simulink model "piezo_constraint"  (R2021a)
settings: Solver=ode1  StartTime=0.0  StopTime=inf  FixedStep=0.001  RelTol=1e-3
PostLoadFcn:
  | , if any(exist('dsrtsu_mdlpostloadfcn', 'file') ~= 0), dsrtsu_mdlpostloadfcn('Execute', bdroot); end,
InitFcn:
  | , if any(exist('rtifpga_mdlclblib', 'file') ~= 0), rtifpga_mdlclblib('Init', bdroot); end,
libraries: simulink x3, rti1202lib_adc_class1 x2, rti1202lib_dac_class1 x1
Description:
  | Standard RTI1202 template.
  | Supported MATLAB version:  R2021a.
settings Model: Tag=RTI1202  DSRTSU_INTERNAL_RTI_VER=610  DSRTSU_INTERNAL_RTI_TYPE=rti1202  RTICANMMDATA=struct('GeneralSetupData',struct('modelroot','C:\Users\VM-User\Desktop\MigrationScripts','generalsettings',struct('filesettings',struct('destfolder',struct('Name','RTICANMM_FILES','Check',1),'buildfolder',struct('Name','.','Check',1),'AbsDestfolder',struct('Name','C:\Users\VM-User\Desktop\MigrationScripts\RTICANMM_FILES'),'AbsBuildfolder',struct('Name','C:\Users\VM-User\Desktop\MigrationScripts'))),'options',struct('addpaths',1,'rmpaths',1,'addtrcexclusion',true,'cannavigator',struct('checkmonitoring',0),'show_usrtrc',0,'use_usrtrc',0),'advanced',struct('options',ones(1,100)),'MPSetup',{{}},'RTI',struct('Type','RTI1202','Ver','7.17','Date','02-Nov-2021'),'modelname','','block','untitled'))  DSRTSU_INTERNAL_RTIFPGA=200  DSRTSU_INTERNAL_RTISTBM_VER=22.2  PacingRate=0.010000  Creator=217_03  LastModifiedBy=217_03
settings SolverCC: AlgebraicLoopSolver=TrustRegion
settings DataIOCC: ReturnWorkspaceOutputs=off
settings OptimizationCC: BlockReduction=off  ConditionallyExecuteInputs=off  OptimizeBlockIOStorage=off  BufferReuse=off  GlobalBufferReuse=off  ExpressionFolding=off  LocalBlockOutputs=off  OptimizeDataStoreBuffers=off  BusAssignmentInplaceUpdate=off
settings DebuggingCC: PregeneratedLibrarySubsystemCodeDiagnostic=none  SFMachineParentedDataDiag=warning  ArithmeticOperatorsInVariantConditions=warning
settings HardwareCC: ProdBitPerPointer=32  ProdBitPerSizeT=32  ProdBitPerPtrDiffT=32  ProdLargestAtomicInteger=Integer  ProdEndianess=BigEndian  ProdWordSize=32  ProdLongLongMode=on  ProdHWDeviceType=Custom Processor->Custom  TargetIntDivRoundTo=Zero  TargetEndianess=BigEndian  TargetHWDeviceType=Custom Processor->Custom
settings ModelReferenceCC: EnableParallelModelReferenceBuilds=on  ParallelModelReferenceMATLABWorkerInit=Load Top Model
settings SFSimCC: SimUseLocalCustomCode=off  MATLABDynamicMemAlloc=off  CustomCodeUndefinedFunction=UseInterfaceOnly
settings RTWCC: Description=dSPACE DS1202 Hardware Platform  SystemTargetFile=rti1202.tlc  MakeCommand=make_rti  TemplateMakefile=rti1202.tmf  RTWUseLocalCustomCode=off
settings CodeAppCC: StateflowObjectComments=on
settings STFCustomTargetCC: ParMdlRefBuildCompliant=on  GRTInterface=off  UseToolchainInfoCompliant=off  SystemTargetFile=rti1202.tlc
settings GRTTargetCC: TargetLangStandard=C89/C90 (ANSI)  CompOptLevelCompliant=off  ConcurrentExecutionCompliant=off  CombineOutputUpdateFcns=off  MatFileLogging=off  CPPClassGenCompliant=off  UseToolchainInfoCompliant=off
settings ConfigComp: CovMetricSettings=dswe

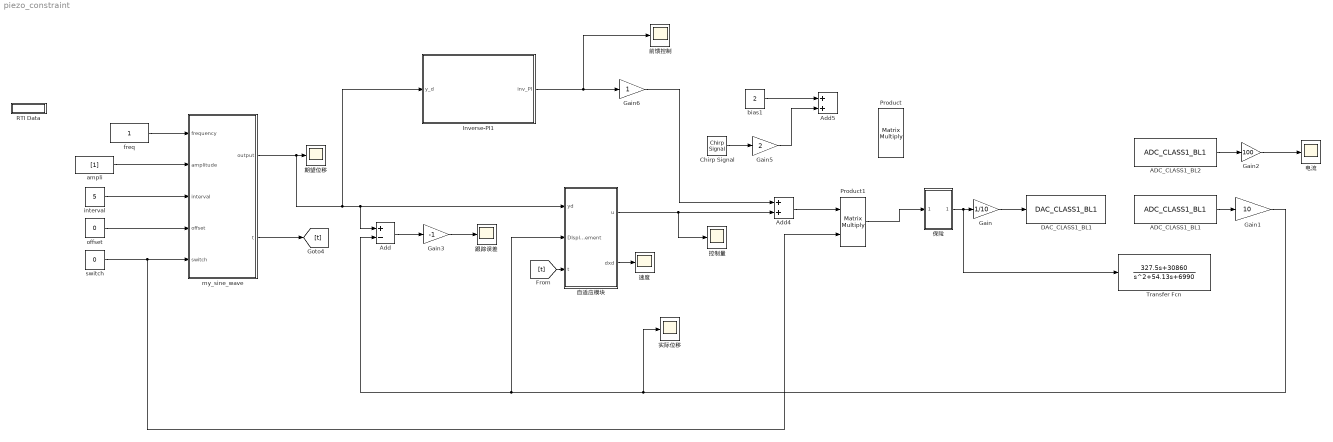
== system piezo_constraint ==
  ADC_CLASS1_BL1 : rti1202lib_adc_class1/ADC_CLASS1_BL1  DSProperties=struct('RTI',struct('Version',uint32(1),'BlockType',struct('isSLSource',uint8(1),'isSLSink',uint8(1),'isHWSource',uint8(0),'isHWSink',uint8(1),'isSetup',uint8(0),'isInline',uint8(1),'isNonInline',uint8(0),'isInterrupt',uint8(0),'isChannelwise',uint8(1)),'IOBoardType',{{'DS120X','STD','ADCC1'}},'UnitType','ADC','Identifier','ADC','DialogType','ML','BlockSet','NONE','SlaveProcessor','NONE'))  RTIBlockInterface=struct('InputPortsActive',0,'InputPortsWidth',int32(1),'InputPortsDataType',{{'SS_BOOLEAN'}},'InputPortsName',{{'Continue'}},'OutputPortsActive',[1 0],'OutputPortsWidth',int32([1 1]),'OutputPortsDataType',{{'SS_DOUBLE','SS_INT16'}},'OutputPortsName',{{'ADC','Status'}},'DialogFcn','rti120xstdadcc1adcgui','SampleTime',{{-1}},'InitLevel',3,'IconTransparency','on','BlockDisplay',{{['ADC CL1\nChannel: 10'],'center'}},'BlockName',struct('Token',{{'ADC_CLASS1_BL1'}}))  RTIBlockParameters=struct('ReadMode',{{1,'OFF',[1 2]}},'ChannelNo',{{10,'OFF',[]}},'ConversionMode',{{1,'OFF',[1 2]}},'TriggerSource',{{1,'OFF',[1 2]}},'TriggerLineIn',{{1,'OFF',[1 16]}},'SampleMode',{{1,'OFF',[1 2]}},'BurstTriggerSource',{{1,'OFF',[1 2]}},'BurstTriggerLine',{{1,'OFF',[1 16]}},'ConvTriggerSource',{{3,'OFF',[1 3]}},'ConvTriggerLine',{{1,'OFF',[1 16]}},'ConvPeriod',{{'100e-6','OFF',[1e-6 1.34]}},'ConvPeriodCheck',{{0,'OFF',[]}},'BurstSize',{{'10','OFF',[]}},'BurstSizeCheck',{{0,'OFF',[]}},'DataSetOffset',{{'0','OFF',[]}},'DataSetOffsetCheck',{{0,'OFF',[]}},'DataSetLength',{{'1','OFF',[]}},'DataSetLengthCheck',{{0,'OFF',[]}},'EnableTriggerEvent',{{0,'OFF',[0 1]}},'TriggerMode',{{2,'OFF',[1 3]}},'TriggerLineOut',{{1,'OFF',[1 16]}},'ADCSWStartEnable',{{0,'OFF',[0 1]}},'SampleTime',{{'-1','OFF',[-1 inf]}},'SampleTimeCheck',{{1,'OFF',[]}},'StatusPortEnable',{{0,'OFF',[0 1]}},'TLCFileName',{{'rti120xadc_c1_adc','OFF',[]}})  RTISFcnParameters=struct('ReadMode','int16','ChannelNo','int16','ConversionMode','int16','TriggerSource','int16','TriggerLineIn','int16','SampleMode','int16','BurstTriggerSource','int16','BurstTriggerLine','int16','ConvTriggerSource','int16','ConvTriggerLine','int16','ConvPeriod','double','BurstSize','int16','DataSetOffset','int16','DataSetLength','int16','EnableTriggerEvent','int16','TriggerMode','int16','TriggerLineOut','int16','ADCSWStartEnable','int16','SampleTime','double','StatusPortEnable','int16','TLCFileName','char')  RTIBlockParaDefault=struct('ReadMode',1,'ChannelNo',1,'ConversionMode',1,'TriggerSource',1,'TriggerLineIn',1,'SampleMode',1,'BurstTriggerSource',1,'BurstTriggerLine',1,'ConvTriggerSource',3,'ConvTriggerLine',1,'ConvPeriod',0.0001,'ConvPeriodCheck',0,'BurstSize',10,'BurstSizeCheck',0,'DataSetOffset',0,'DataSetOffsetCheck',0,'DataSetLength',1,'DataSetLengthCheck',0,'EnableTriggerEvent',0,'TriggerMode',2,'TriggerLineOut',1,'ADCSWStartEnable',0,'SampleTime',-1,'SampleTimeCheck',1,'StatusPortEnable',0,'TLCFileName','rti120xadc_c1_adc')
  ADC_CLASS1_BL2 : rti1202lib_adc_class1/ADC_CLASS1_BL1  DSProperties=struct('RTI',struct('Version',uint32(1),'BlockType',struct('isSLSource',uint8(1),'isSLSink',uint8(1),'isHWSource',uint8(0),'isHWSink',uint8(1),'isSetup',uint8(0),'isInline',uint8(1),'isNonInline',uint8(0),'isInterrupt',uint8(0),'isChannelwise',uint8(1)),'IOBoardType',{{'DS120X','STD','ADCC1'}},'UnitType','ADC','Identifier','ADC','DialogType','ML','BlockSet','NONE','SlaveProcessor','NONE'))  RTIBlockInterface=struct('InputPortsActive',0,'InputPortsWidth',int32(1),'InputPortsDataType',{{'SS_BOOLEAN'}},'InputPortsName',{{'Continue'}},'OutputPortsActive',[1 0],'OutputPortsWidth',int32([1 1]),'OutputPortsDataType',{{'SS_DOUBLE','SS_INT16'}},'OutputPortsName',{{'ADC','Status'}},'DialogFcn','rti120xstdadcc1adcgui','SampleTime',{{-1}},'InitLevel',3,'IconTransparency','on','BlockDisplay',{{['ADC CL1\nChannel: 13'],'center'}},'BlockName',struct('Token',{{'ADC_CLASS1_BL1'}}))  RTIBlockParameters=struct('ReadMode',{{1,'OFF',[1 2]}},'ChannelNo',{{13,'OFF',[]}},'ConversionMode',{{1,'OFF',[1 2]}},'TriggerSource',{{1,'OFF',[1 2]}},'TriggerLineIn',{{1,'OFF',[1 16]}},'SampleMode',{{1,'OFF',[1 2]}},'BurstTriggerSource',{{1,'OFF',[1 2]}},'BurstTriggerLine',{{1,'OFF',[1 16]}},'ConvTriggerSource',{{3,'OFF',[1 3]}},'ConvTriggerLine',{{1,'OFF',[1 16]}},'ConvPeriod',{{'100e-6','OFF',[1e-6 1.34]}},'ConvPeriodCheck',{{0,'OFF',[]}},'BurstSize',{{'10','OFF',[]}},'BurstSizeCheck',{{0,'OFF',[]}},'DataSetOffset',{{'0','OFF',[]}},'DataSetOffsetCheck',{{0,'OFF',[]}},'DataSetLength',{{'1','OFF',[]}},'DataSetLengthCheck',{{0,'OFF',[]}},'EnableTriggerEvent',{{0,'OFF',[0 1]}},'TriggerMode',{{2,'OFF',[1 3]}},'TriggerLineOut',{{1,'OFF',[1 16]}},'ADCSWStartEnable',{{0,'OFF',[0 1]}},'SampleTime',{{'-1','OFF',[-1 inf]}},'SampleTimeCheck',{{1,'OFF',[]}},'StatusPortEnable',{{0,'OFF',[0 1]}},'TLCFileName',{{'rti120xadc_c1_adc','OFF',[]}})  RTISFcnParameters=struct('ReadMode','int16','ChannelNo','int16','ConversionMode','int16','TriggerSource','int16','TriggerLineIn','int16','SampleMode','int16','BurstTriggerSource','int16','BurstTriggerLine','int16','ConvTriggerSource','int16','ConvTriggerLine','int16','ConvPeriod','double','BurstSize','int16','DataSetOffset','int16','DataSetLength','int16','EnableTriggerEvent','int16','TriggerMode','int16','TriggerLineOut','int16','ADCSWStartEnable','int16','SampleTime','double','StatusPortEnable','int16','TLCFileName','char')  RTIBlockParaDefault=struct('ReadMode',1,'ChannelNo',1,'ConversionMode',1,'TriggerSource',1,'TriggerLineIn',1,'SampleMode',1,'BurstTriggerSource',1,'BurstTriggerLine',1,'ConvTriggerSource',3,'ConvTriggerLine',1,'ConvPeriod',0.0001,'ConvPeriodCheck',0,'BurstSize',10,'BurstSizeCheck',0,'DataSetOffset',0,'DataSetOffsetCheck',0,'DataSetLength',1,'DataSetLengthCheck',0,'EnableTriggerEvent',0,'TriggerMode',2,'TriggerLineOut',1,'ADCSWStartEnable',0,'SampleTime',-1,'SampleTimeCheck',1,'StatusPortEnable',0,'TLCFileName','rti120xadc_c1_adc')
  Add : Sum  Inputs=+-
  Add4 : Sum
  Add5 : Sum
  Chirp Signal : simulink/Sources/Chirp Signal  f1=1  T=20  f2=50
  DAC_CLASS1_BL1 : rti1202lib_dac_class1/DAC_CLASS1_BL1  DSProperties=struct('RTI',struct('Version',uint32(2),'BlockType',struct('isSLSource',uint8(0),'isSLSink',uint8(1),'isHWSource',uint8(0),'isHWSink',uint8(1),'isSetup',uint8(0),'isInline',uint8(1),'isNonInline',uint8(0),'isInterrupt',uint8(0),'isChannelwise',uint8(1)),'IOBoardType',{{'DS120X','STD','DACC1'}},'UnitType','DAC','Identifier','DAC','DialogType','ML','BlockSet','NONE','SlaveProcessor','NONE'))  RTIBlockInterface=struct('InputPortsActive',1,'InputPortsWidth',int32(1),'InputPortsDataType',{{'SS_DOUBLE'}},'InputPortsName',{{['DAC 5']}},'DialogFcn','rti120xstddacc1dacgui','InitLevel',3,'IconTransparency','on','BlockDisplay',{{['DAC CL1\nChannel: 5'],'center'}},'BlockName',struct('Token',{{'DAC_CLASS1_BL1'}}))  RTIBlockParameters=struct('ChannelNo',{{5,'OFF',[]}},'ChannelNumOf',{{1,'OFF',[]}},'InitialValue1',{{'0','OFF',[-10 10]}},'InitialValue2',{{'0','OFF',[-10 10]}},'InitialValue3',{{'0','OFF',[-10 10]}},'InitialValue4',{{'0','OFF',[-10 10]}},'InitialValue5',{{'0','OFF',[-10 10]}},'InitialValue6',{{'0','OFF',[-10 10]}},'InitialValue7',{{'0','OFF',[-10 10]}},'InitialValue8',{{'0','OFF',[-10 10]}},'InitialValue9',{{'0','OFF',[-10 10]}},'InitialValue10',{{'0','OFF',[-10 10]}},'InitialValue11',{{'0','OFF',[-10 10]}},'InitialValue12',{{'0','OFF',[-10 10]}},'InitialValue13',{{'0','OFF',[-10 10]}},'InitialValue14',{{'0','OFF',[-10 10]}},'InitialValue15',{{'0','OFF',[-10 10]}},'InitialValue16',{{'0','OFF',[-10 10]}},'OutputMode',{{ones(1,16),'OFF',[1 2]}},'TermValue1',{{'0','OFF',[-10 10]}},'TermValue2',{{'0','OFF',[-10 10]}},'TermValue3',{{'0','OFF',[-10 10]}},'TermValue4',{{'0','OFF',[-10 10]}},'TermValue5',{{'0','OFF',[-10 10]}},'TermValue6',{{'0','OFF',[-10 10]}},'TermValue7',{{'0','OFF',[-10 10]}},'TermValue8',{{'0','OFF',[-10 10]}},'TermValue9',{{'0','OFF',[-10 10]}},'TermValue10',{{'0','OFF',[-10 10]}},'TermValue11',{{'0','OFF',[-10 10]}},'TermValue12',{{'0','OFF',[-10 10]}},'TermValue13',{{'0','OFF',[-10 10]}},'TermValue14',{{'0','OFF',[-10 10]}},'TermValue15',{{'0','OFF',[-10 10]}},'TermValue16',{{'0','OFF',[-10 10]}},'EnableTermMode',{{0,'OFF',[0 1]}},'TLCFileName',{{'rti120xdac_c1_dac','OFF',[]}},'InitialValueBuildCheck1',{{0,'OFF',[]}},'InitialValueBuildCheck2',{{0,'OFF',[]}},'InitialValueBuildCheck3',{{0,'OFF',[]}},'InitialValueBuildCheck4',{{0,'OFF',[]}},'InitialValueBuildCheck5',{{1,'OFF',[]}},'InitialValueBuildCheck6',{{0,'OFF',[]}},'InitialValueBuildCheck7',{{0,'OFF',[]}},'InitialValueBuildCheck8',{{0,'OFF',[]}},'InitialValueBuildCheck9',{{0,'OFF',[]}},'InitialValueBuildCheck10',{{0,'OFF',[]}},'InitialValueBuildCheck11',{{0,'OFF',[]}},'InitialValueBuildCheck12',{{0,'OFF',[]}},'InitialValueBuildCheck13',{{0,'OFF',[]}},'InitialValueBuildCheck14',{{0,'OFF',[]}},'InitialValueBuildCheck15',{{0,'OFF',[]}},'InitialValueBuildCheck16',{{0,'OFF',[]}},'TermValueBuildCheck1',{{0,'OFF',[]}},'TermValueBuildCheck2',{{0,'OFF',[]}},'TermValueBuildCheck3',{{0,'OFF',[]}},'TermValueBuildCheck4',{{0,'OFF',[]}},'TermValueBuildCheck5',{{0,'OFF',[]}},'TermValueBuildCheck6',{{0,'OFF',[]}},'TermValueBuildCheck7',{{0,'OFF',[]}},'TermValueBuildCheck8',{{0,'OFF',[]}},'TermValueBuildCheck9',{{0,'OFF',[]}},'TermValueBuildCheck10',{{0,'OFF',[]}},'TermValueBuildCheck11',{{0,'OFF',[]}},'TermValueBuildCheck12',{{0,'OFF',[]}},'TermValueBuildCheck13',{{0,'OFF',[]}},'TermValueBuildCheck14',{{0,'OFF',[]}},'TermValueBuildCheck15',{{0,'OFF',[]}},'TermValueBuildCheck16',{{0,'OFF',[]}})  RTISFcnParameters=struct('ChannelNo','int16','ChannelNumOf','int16','InitialValue1','double','InitialValue2','double','InitialValue3','double','InitialValue4','double','InitialValue5','double','InitialValue6','double','InitialValue7','double','InitialValue8','double','InitialValue9','double','InitialValue10','double','InitialValue11','double','InitialValue12','double','InitialValue13','double','InitialValue14','double','InitialValue15','double','InitialValue16','double','OutputMode','int16','TermValue1','double','TermValue2','double','TermValue3','double','TermValue4','double','TermValue5','double','TermValue6','double','TermValue7','double','TermValue8','double','TermValue9','double','TermValue10','double','TermValue11','double','TermValue12','double','TermValue13','double','TermValue14','double','TermValue15','double','TermValue16','double','EnableTermMode','int16','TLCFileName','char')  RTIBlockParaDefault=struct('ChannelNo',1,'ChannelNumOf',1,'InitialValue1',0,'InitialValue2',0,'InitialValue3',0,'InitialValue4',0,'InitialValue5',0,'InitialValue6',0,'InitialValue7',0,'InitialValue8',0,'InitialValue9',0,'InitialValue10',0,'InitialValue11',0,'InitialValue12',0,'InitialValue13',0,'InitialValue14',0,'InitialValue15',0,'InitialValue16',0,'OutputMode',ones(1,16),'TermValue1',0,'TermValue2',0,'TermValue3',0,'TermValue4',0,'TermValue5',0,'TermValue6',0,'TermValue7',0,'TermValue8',0,'TermValue9',0,'TermValue10',0,'TermValue11',0,'TermValue12',0,'TermValue13',0,'TermValue14',0,'TermValue15',0,'TermValue16',0,'EnableTermMode',0,'TLCFileName','rti120xdac_c1_dac','InitialValueBuildCheck1',0,'InitialValueBuildCheck2',0,'InitialValueBuildCheck3',0,'InitialValueBuildCheck4',0,'InitialValueBuildCheck5',0,'InitialValueBuildCheck6',0,'InitialValueBuildCheck7',0,'InitialValueBuildCheck8',0,'InitialValueBuildCheck9',0,'InitialValueBuildCheck10',0,'InitialValueBuildCheck11',0,'InitialValueBuildCheck12',0,'InitialValueBuildCheck13',0,'InitialValueBuildCheck14',0,'InitialValueBuildCheck15',0,'InitialValueBuildCheck16',0,'TermValueBuildCheck1',0,'TermValueBuildCheck2',0,'TermValueBuildCheck3',0,'TermValueBuildCheck4',0,'TermValueBuildCheck5',0,'TermValueBuildCheck6',0,'TermValueBuildCheck7',0,'TermValueBuildCheck8',0,'TermValueBuildCheck9',0,'TermValueBuildCheck10',0,'TermValueBuildCheck11',0,'TermValueBuildCheck12',0,'TermValueBuildCheck13',0,'TermValueBuildCheck14',0,'TermValueBuildCheck15',0,'TermValueBuildCheck16',0)
  Gain : Gain  Gain=1/10
  Gain1 : Gain  Gain=10
  Gain2 : Gain  Gain=100
  Gain3 : Gain  Gain=-1
  Gain5 : Gain  Gain=2
  Gain6 : Gain
  Inverse-PI1 : Subsystem
  Product : Product  Multiplication=Matrix(*)  OutDataTypeStr=double
  Product1 : Product  Multiplication=Matrix(*)  OutDataTypeStr=double
  RTI Data : Subsystem  Tag=struct('RTIDataServer',struct('RTIDataServerVs','2','RTIModelDescription','struct(''main'',''piezo_constraint_huheyu'',''sub'','''',''isMp'',0)'))  LoadFcn="if exist('rtidc'), try,  rtidc('DataHostBlockClbLoad', gcbh); catch, disp(['Warning: ''LoadFcn'' for RTI Data block failed: ' lasterr]); end, end,"  mask(RTI_DATA_HOST){}
      mask help:
      | RTI Data Block.
      | This block is used by RTI to store internal model-dependent data.
      | Please keep this block on the root level of the model. Deleting this block will result in data loss.
      |
      | NEVER DELETE OR COPY THIS BLOCK!
      settings: CopyFcn="if exist('rtidc'), try,  rtidc('DataHostBlockClbCopy', gcbh); catch, disp(['Warning: ''CopyFcn'' for RTI Data block failed: ' lasterr]); end, end,"  DeleteFcn="if exist('rtidc'), try,  rtidc('DataHostBlockClbDelete', gcbh); catch, disp(['Warning: ''DeleteFcn'' for RTI Data block failed: ' lasterr]); end, end,"  ModelCloseFcn="if exist('rtidc'), try,  rtidc('DataHostBlockClbModelClose', gcbh); catch, disp(['Warning: ''ModelCloseFcn'' for RTI Data block failed: ' lasterr]); end, end,"  PreSaveFcn="if exist('rtidc'), try,  rtidc('DataHostBlockClbPreSave', gcbh); catch, disp(['Warning: ''PreSaveFcn'' for RTI Data block failed: ' lasterr]); end, end,"  PostSaveFcn="if exist('rtidc'), try,  rtidc('DataHostBlockClbPostSave', gcbh); catch, disp(['Warning: ''PostSaveFcn'' for RTI Data block failed: ' lasterr]); end, end,"  NameChangeFcn="if exist('rtidc'), try,  rtidc('DataHostBlockClbNameChange', gcbh); catch, disp(['Warning: ''NameChangeFcn'' for RTI Data block failed: ' lasterr]); end, end,"
      mask Help:
      | RTI Data Block.
      | This block is used by RTI to store internal model-dependent data.
      | Please keep this block on the root level of the model. Deleting this block will result in data loss.
      | 
      | NEVER DELETE OR COPY THIS BLOCK!
      mask Display:
      | text(0.5, 0.5, 'RTI Data', 'HorizontalAlignment', 'center');
      | plot([1 0]);
  Transfer Fcn : TransferFcn  Numerator=[327.5 30860]  Denominator=[1 54.13 6990]
  ampli : Constant  Value=[1]
  bias1 : Constant  Value=2
  freq : Constant
  interval : Constant  Value=5
  my_sine_wave : Subsystem
  offset : Constant  Value=0
  switch : Constant  Value=0  OutMin=[0]  OutMax=[1]  OutDataTypeStr=int8
  保险 : Subsystem
  前馈控制 : Scope
  实际位移 : Scope
  控制量 : Scope
  期望位移 : Scope
  电流 : Scope
  自适应模块 : Subsystem
  跟踪误差 : Scope
  速度 : Scope
  wires:
  ampli/1 -> my_sine_wave/2(amplitude)
  interval/1 -> my_sine_wave/3(interval)
  ADC_CLASS1_BL1/1 -> Gain1/1
  Gain/1 -> DAC_CLASS1_BL1/1
  保险/1(Out2) -> Transfer Fcn/1, Gain/1
  my_sine_wave/1(output) -> Inverse-PI1/1(y_d), 自适应模块/1(yd), Add/1, 期望位移/1
  ADC_CLASS1_BL2/1 -> Gain2/1
  Gain2/1 -> 电流/1
  Inverse-PI1/1(inv_PI) -> 前馈控制/1, Gain6/1
  Chirp Signal/1 -> Gain5/1
  bias1/1 -> Add5/1
  Gain5/1 -> Add5/2
  Gain6/1 -> Add4/1
  my_sine_wave/2(t) -> [t]
  switch/1 -> Product1/2, my_sine_wave/5(switch)
  offset/1 -> my_sine_wave/4(offset)
  freq/1 -> my_sine_wave/1(frequency)
  Product1/1 -> 保险/1(In1)
  自适应模块/1(u) -> 控制量/1, Add4/2
  Add4/1 -> Product1/1
  [t] -> 自适应模块/3(t)
  Gain1/1 -> 实际位移/1, 自适应模块/2(DIsplacement), Add/2
  Gain3/1 -> 跟踪误差/1
  Add/1 -> Gain3/1
  自适应模块/2(dxd) -> 速度/1

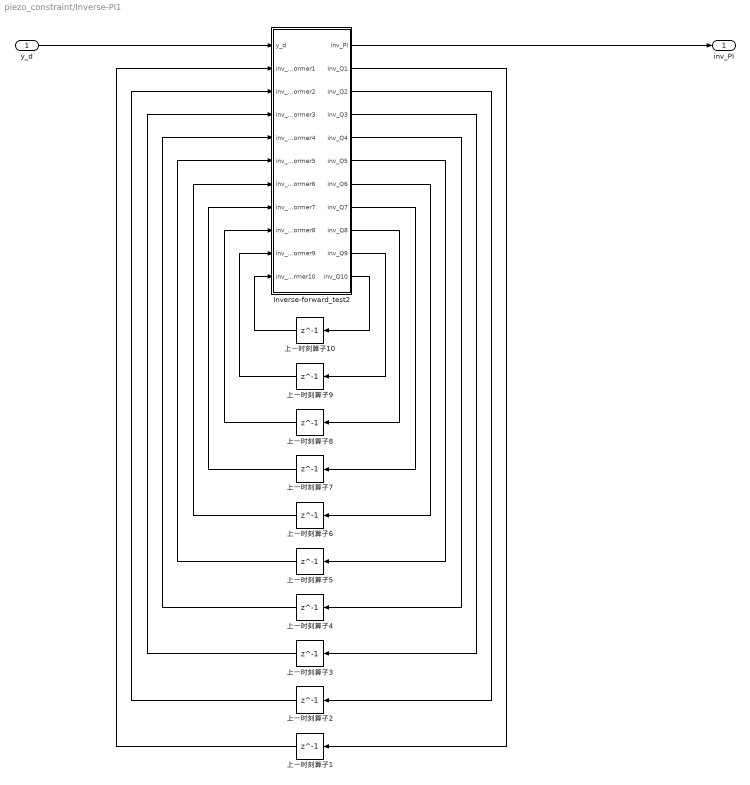
== system piezo_constraint/Inverse-PI1 ==
  y_d : Inport
  Inverse-forward_test2 : MATLAB Function  TreatAsAtomicUnit=on
  上一时刻算子{1..10} (10 alike) : Delay  DelayLength=1
  inv_PI : Outport
  wires:
  Inverse-forward_test2/1(inv_PI) -> inv_PI/1
  y_d/1 -> Inverse-forward_test2/1(y_d)
  Inverse-forward_test2/8(inv_Q7) -> 上一时刻算子7/1
  Inverse-forward_test2/10(inv_Q9) -> 上一时刻算子9/1
  上一时刻算子3/1 -> Inverse-forward_test2/4(inv_Q_former3)
  上一时刻算子9/1 -> Inverse-forward_test2/10(inv_Q_former9)
  Inverse-forward_test2/3(inv_Q2) -> 上一时刻算子2/1
  Inverse-forward_test2/6(inv_Q5) -> 上一时刻算子5/1
  Inverse-forward_test2/4(inv_Q3) -> 上一时刻算子3/1
  Inverse-forward_test2/5(inv_Q4) -> 上一时刻算子4/1
  Inverse-forward_test2/2(inv_Q1) -> 上一时刻算子1/1
  上一时刻算子8/1 -> Inverse-forward_test2/9(inv_Q_former8)
  Inverse-forward_test2/11(inv_Q10) -> 上一时刻算子10/1
  上一时刻算子6/1 -> Inverse-forward_test2/7(inv_Q_former6)
  Inverse-forward_test2/7(inv_Q6) -> 上一时刻算子6/1
  上一时刻算子10/1 -> Inverse-forward_test2/11(inv_Q_former10)
  上一时刻算子7/1 -> Inverse-forward_test2/8(inv_Q_former7)
  上一时刻算子1/1 -> Inverse-forward_test2/2(inv_Q_former1)
  上一时刻算子4/1 -> Inverse-forward_test2/5(inv_Q_former4)
  上一时刻算子5/1 -> Inverse-forward_test2/6(inv_Q_former5)
  Inverse-forward_test2/9(inv_Q8) -> 上一时刻算子8/1
  上一时刻算子2/1 -> Inverse-forward_test2/3(inv_Q_former2)

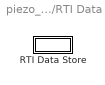
== system piezo_constraint/RTI Data ==
  RTI Data Store : Subsystem  Tag="struct('public',struct('sub',struct('name',{{'piezo_constraint_huheyu'}},'data',{{struct('TH',struct('thTaskInfo',struct('taskType',{'TIMER','HWINT','TMRINT','SWINT','GLINT'},'tasksNumOf',{1,0,0,0,0},'srcIds',{{'TIMERA'},{},{},{},{}},'taskNames',{{['Timer Task 1']},{},{},{},{}})),'th_tc',struct('dataType','TASK','taskGroupId','','taskGroupList',{{}},'taskSchedulingPolicy','FCFS','taskType','TIMER','blkh',-1,'srcId','TIMERA','srcSgnName',['Timer A interrupt'],'srcCpuName','','taskName',['Timer Task 1  [0.001] s'],'taskNameDisplayExt','','smplTime',0.001,'smplTimeOffs',0,'hasFixedPriority',0,'priority',1,'hasFixedOvc',0,'ovcType',1,'ovcMax',1),'tc_th',struct('dataType','TASK','taskGroupId','','taskGroupList',{{}},'taskSchedulingPolicy','FCFS','taskType','TIMER','blkh',-1,'srcId','TIMERA','srcSgnName',['Timer A interrupt'],'srcCpuName','','taskName',['Timer Task 1  [0.001] s'],'taskNameDisplayExt','','smplTime',0.001,'smplTimeOffs',0,'hasFixedPriority',0,'priority',1,'hasFixedOvc',0,'ovcType',1,'ovcMax',1))}})),'private',struct('version',struct('dsVer',uint32(2)),'access',struct('modified',['19-Jan-2024 18:22:50'],'type','Model','isPerm',1)))"  mask(RTI_DATA_STORE){}
      mask help:
      | RTI Data Store Block. This block is used by RTI to store internal model dependent data. Deleting this block will result in data loss.
      |
      | NEVER DELETE, COPY, OR MODIFY THIS BLOCK!
      mask Help:
      | RTI Data Store Block. This block is used by RTI to store internal model dependent data. Deleting this block will result in data loss.
      | 
      | NEVER DELETE, COPY, OR MODIFY THIS BLOCK!
      mask Display: text(0.5, 0.5, ' ', 'HorizontalAlignment', 'center');

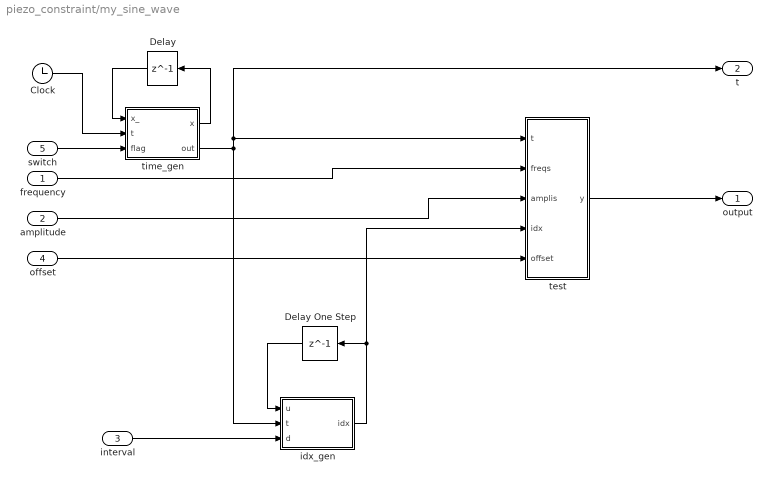
== system piezo_constraint/my_sine_wave ==
  frequency : Inport
  amplitude : Inport  Port=2
  interval : Inport  Port=3
  offset : Inport  Port=4
  switch : Inport  Port=5
  Clock : Clock
      settings: Decimation=100
  Delay : Delay  DelayLength=1
  Delay One Step : Delay  DelayLength=1  InitialCondition=0
  idx_gen : MATLAB Function  TreatAsAtomicUnit=on
  test : MATLAB Function  TreatAsAtomicUnit=on
  time_gen : MATLAB Function  TreatAsAtomicUnit=on
  output : Outport
  t : Outport  Port=2
  wires:
  idx_gen/1(idx) -> Delay One Step/1, test/4(idx)
  test/1(y) -> output/1
  Delay One Step/1 -> idx_gen/1(u)
  frequency/1 -> test/2(freqs)
  amplitude/1 -> test/3(amplis)
  interval/1 -> idx_gen/3(d)
  Clock/1 -> time_gen/2(t)
  time_gen/2(out) -> idx_gen/2(t), t/1, test/1(t)
  switch/1 -> time_gen/3(flag)
  time_gen/1(x) -> Delay/1
  Delay/1 -> time_gen/1(x_)
  offset/1 -> test/5(offset)

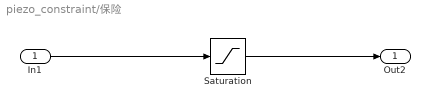
== system piezo_constraint/保险 ==
  In1 : Inport
  Saturation : Saturate  UpperLimit=5  LowerLimit=-5  OutDataTypeStr=double
  Out2 : Outport
  wires:
  Saturation/1 -> Out2/1
  In1/1 -> Saturation/1

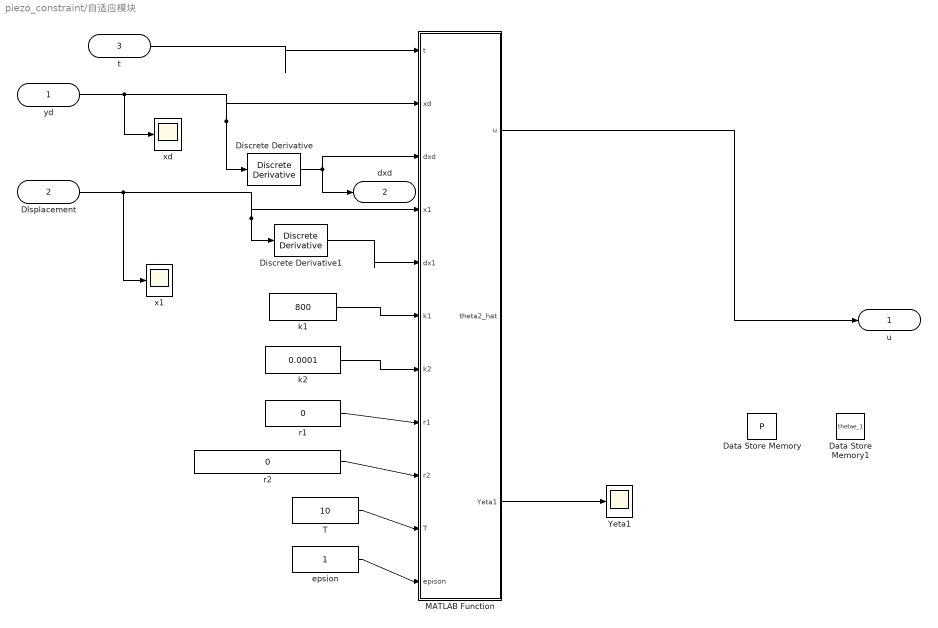
== system piezo_constraint/自适应模块 ==
  yd : Inport
  DIsplacement : Inport  Port=2
  t : Inport  Port=3
  Data Store Memory : DataStoreMemory  DataStoreName=P  ReadBeforeWriteMsg=warning  WriteAfterWriteMsg=warning  WriteAfterReadMsg=warning  InitialValue=0*eye(4)  ShowAdditionalParam=off  OutDataTypeStr=double
  Data Store Memory1 : DataStoreMemory  DataStoreName=thetae_1  ReadBeforeWriteMsg=warning  WriteAfterWriteMsg=warning  WriteAfterReadMsg=warning  InitialValue=[1;1;1;1]*0  ShowAdditionalParam=off  OutDataTypeStr=double
  Discrete Derivative : simulink/Discrete/Discrete Derivative  gainval=1  ICPrevScaledInput=0.0  OutMin=[]  OutMax=[]  OutDataType=fixdt(1, 16)  OutScaling=2^-10  DoSatur=off
  Discrete Derivative1 : simulink/Discrete/Discrete Derivative  gainval=1  ICPrevScaledInput=0.0  OutMin=[]  OutMax=[]  OutDataType=fixdt(1, 16)  OutScaling=2^-10  DoSatur=off
  MATLAB Function : MATLAB Function  TreatAsAtomicUnit=on
  T : Constant  Value=10
  Yeta1 : Scope
  epsion : Constant
  k1 : Constant  Value=800
  k2 : Constant  Value=0.0001
  r1 : Constant  Value=0
  r2 : Constant  Value=0
  x1 : Scope
  xd : Scope
  u : Outport
  dxd : Outport  Port=2
  wires:
  DIsplacement/1 -> x1/1, Discrete Derivative1/1, MATLAB Function/4(x1)
  MATLAB Function/1(u) -> u/1
  yd/1 -> xd/1, MATLAB Function/2(xd), Discrete Derivative/1
  Discrete Derivative/1 -> MATLAB Function/3(dxd), dxd/1
  Discrete Derivative1/1 -> MATLAB Function/5(dx1)
  k1/1 -> MATLAB Function/6(k1)
  k2/1 -> MATLAB Function/7(k2)
  r1/1 -> MATLAB Function/8(r1)
  r2/1 -> MATLAB Function/9(r2)
  t/1 -> MATLAB Function/1(t)
  epsion/1 -> MATLAB Function/11(epison)
  T/1 -> MATLAB Function/10(T)
  MATLAB Function/3(Yeta1) -> Yeta1/1

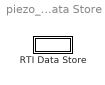
== system piezo_constraint/RTI Data/RTI Data Store ==
  RTI Data Store : Subsystem  mask(RTI_DATA_STORE){}
      mask help:
      | RTI Data Store Block. This block is used by RTI to store internal model dependent data. Deleting this block will result in data loss.
      |
      | NEVER DELETE, COPY, OR MODIFY THIS BLOCK!
      mask Help:
      | RTI Data Store Block. This block is used by RTI to store internal model dependent data. Deleting this block will result in data loss.
      | 
      | NEVER DELETE, COPY, OR MODIFY THIS BLOCK!
      mask Display: text(0.5, 0.5, ' ', 'HorizontalAlignment', 'center');

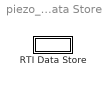
== system piezo_constraint/RTI Data/RTI Data Store/RTI Data Store ==
  RTI Data Store : Subsystem  mask(RTI_DATA_STORE){}
      mask help:
      | RTI Data Store Block. This block is used by RTI to store internal model dependent data. Deleting this block will result in data loss.
      |
      | NEVER DELETE, COPY, OR MODIFY THIS BLOCK!
      mask Help:
      | RTI Data Store Block. This block is used by RTI to store internal model dependent data. Deleting this block will result in data loss.
      | 
      | NEVER DELETE, COPY, OR MODIFY THIS BLOCK!
      mask Display: text(0.5, 0.5, ' ', 'HorizontalAlignment', 'center');

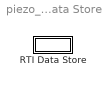
== system piezo_constraint/RTI Data/RTI Data Store/RTI Data Store/RTI Data Store ==
  RTI Data Store : Subsystem  mask(RTI_DATA_STORE){}
      mask help:
      | RTI Data Store Block. This block is used by RTI to store internal model dependent data. Deleting this block will result in data loss.
      |
      | NEVER DELETE, COPY, OR MODIFY THIS BLOCK!
      mask Help:
      | RTI Data Store Block. This block is used by RTI to store internal model dependent data. Deleting this block will result in data loss.
      | 
      | NEVER DELETE, COPY, OR MODIFY THIS BLOCK!
      mask Display: text(0.5, 0.5, ' ', 'HorizontalAlignment', 'center');

== system piezo_constraint/RTI Data/RTI Data Store/RTI Data Store/RTI Data Store/RTI Data Store ==

== matlab function piezo_constraint/自适应模块/MATLAB Function ==
  settings: updateMethod=DISCRETE
  data: t input; xd input; dxd input; x1 input; dx1 input; k1 input; k2 input; P data_store_memory; thetae_1 data_store_memory; u output; r1 input; r2 input; theta2_hat output; Yeta1 output; T input; epison input
function [u,theta2_hat,Yeta1]  = myRLS(t,xd,dxd,x1,dx1,k1,k2,r1,r2,T,epison)
% theta = [1.478; - 0.4776;0.51469791;- 0.515080];[1.777;-0.7768;0.2314;0.2313]
%%  最小二乘估计
global P thetae_1;
%lambda = 1;                         %遗忘因子范围[0.9 1]
%phi = [y_1;y_2;u_1;u_2];            %phi为数据向量
%K = P*phi/(lambda+phi'*P*phi);      %K(k+1)时刻的值
%thetae = thetae_1 + K*(y - phi'*thetae_1); %thetae(:,k)
%P = (eye(4)-K*phi')*P/lambda;
%thetae_1 = thetae;                  %thetae(:,k)
% u = (phi'* thetae_1);%/(thetae_1(3));               %  G为估计量的输出
%%  控制信号计算
%phi1 = [y;y_1;0;u_1];               % k时刻的phi
%u = (-phi1'*thetae+yd)/(thetae(3));

%T=20;epison=1;
if t<T
    Yeta1=(1/(t+0.01)-1/T)^3+epison;
    if Yeta1>10
        Yeta1=100;
    end
else
    Yeta1=epison;
end
e=x1-xd;
h11=1-(e/Yeta1)^2;


F1=30;F2=500;
h12=1-(x1/F1)^2;
h2=1-(dx1/F2)^2;
h1=h11*h12/(h11+h12);
%h1=h11;
%h2=1;

ksi1=e/h1;
ksi2=dx1/h2;
%mu1=1;
%mu2=1;
mu1=1/h1;
mu2=1/h2;

z1=ksi1;
ci1=[0 0 0 0]';
xi1=[x1,xd,dx1,dxd]';

fai1=exp(-(xi1-ci1)'*(xi1-ci1)/4);
faic1=fai1*fai1+1;
dtheta1_hat=P(1,2);
theta1_hat_d=P(1,3);
theta1_hat=theta1_hat_d+0.001*dtheta1_hat;
alpha1=1/h2*(-k1*z1+dxd-r1*mu1*theta1_hat*faic1*z1);
dtheta1_hat=-r1*theta1_hat+r1*mu1*mu1*faic1*z1*z1;
P(1,2)=dtheta1_hat;
P(1,3)=theta1_hat;

z2=ksi2-alpha1;
dtheta2_hat=P(2,2);
theta2_hat_d=P(2,3);
theta2_hat=theta2_hat_d+0.001*dtheta2_hat;
dtheta2_hat=-r2*theta2_hat+r2*mu2*mu2*z2*z2*faic1;
P(2,2)=dtheta2_hat;
P(2,3)=theta2_hat_d;
u=-k2*z2-0*1/mu2*mu1*mu1*h2*h2*z1*z1*z2-r2*mu2*theta2_hat*faic1*z2;
%u=-k2*z2-r2*mu2*theta2_hat*faic1*z2;
end
%%  离散 最小二乘估计    
% for k = 3:length(v)
%     phi = [y(k-1);y(k-2);y_PI(k-1);y_PI(k-2)];   %phi为列向量
%     % 递推最小二乘法
%     K = P*phi/(lambda+phi'*P*phi);
%     thetae(:,k) = thetae_1 + K*(y(k)-phi'*thetae_1);
%     P = (eye(4)-K*phi')*P/lambda;
%     % 更新数据
%     thetae_1 = thetae(:,k);
%     G(k) = phi'* thetae_1;
% end

== matlab function piezo_constraint/my_sine_wave/idx_gen ==
  data: u input; idx output; t input; d input
function idx = fcn(u,t,d)
if t == 0
   idx = 1;
else
    if mod(t, d) == 0   %返回用 d 除以 t 后的余数
       idx = u + 1;
    else
       idx = u;
    end
end

== matlab function piezo_constraint/my_sine_wave/test ==
  data: t input; y output; freqs input; amplis input; idx input; offset input
function y = fcn(t,freqs,amplis,idx,offset)
idx = int32(idx);
if idx < length(freqs)
    y = amplis(idx) * cos(2 * pi * freqs(idx) * t)+offset;
else
    y = amplis(end) * cos(2 * pi * freqs(end) * t)+offset;
end

== matlab function piezo_constraint/my_sine_wave/time_gen ==
  data: x_ input; x output; t input; out output; flag input
function [x,out] = fcn(x_,t,flag)
if flag == 0
    x = t + 0.001;
    out = 0;
else
    x = x_;
    out = t - x;
end

== matlab function piezo_constraint/Inverse-PI1/Inverse-forward_test2 ==
  data: y_d input; inv_PI output; inv_Q_former1 input; inv_Q1 output; inv_Q_former2 input; inv_Q_former3 input; inv_Q2 output; inv_Q3 output; inv_Q4 output; inv_Q5 output; inv_Q6 output; inv_Q7 output; inv_Q8 output; inv_Q9 output; inv_Q10 output; inv_Q_former4 input; inv_Q_former5 input; inv_Q_former6 input; inv_Q_former7 input; inv_Q_former8 input; inv_Q_former9 input; inv_Q_former10 input
function [inv_PI,inv_Q1,inv_Q2,inv_Q3,inv_Q4,inv_Q5,inv_Q6,inv_Q7,inv_Q8,inv_Q9,inv_Q10] = fcn(y_d,inv_Q_former1,inv_Q_former2,inv_Q_former3,inv_Q_former4,inv_Q_former5,inv_Q_former6,inv_Q_former7,inv_Q_former8,inv_Q_former9,inv_Q_former10)
%%    导入PI模型的权重
% weigh = [0.311694,0.050216,0.024070,0.015965,0.084121,4.249776e-09,5.7480264e-10,3.640272e-11,1.756862e-12,1.222629];

% inv_weigh = [3.208271,-0.445158,-0.172313,-0.102906,-0.430567,-1.79875e-08,-2.432903e-09,-1.540777e-10,-7.436078e-12,-1.472084];
% inv_threshold = [0,0.748066,1.616652,2.543007,3.507679,4.674242,5.840805,7.0073677,8.1739306,9.3404936 ];
inv_weigh = [1.7312759,-0.358271,-0.0353503,-0.0885164,-0.1784628,-0.02757898,-0.0553805,-0.16352052,-0.1170679,-0.0879477];
inv_threshold = [0,0.1155217,0.261188,0.4107031,0.5708135,0.7576115,0.949348,1.151836,1.394497,1.677331];

inv_Q1 = max(y_d - inv_threshold(1),min(y_d + inv_threshold(1),inv_Q_former1));
inv_Q2 = max(y_d - inv_threshold(2),min(y_d + inv_threshold(2),inv_Q_former2));
inv_Q3 = max(y_d - inv_threshold(3),min(y_d + inv_threshold(3),inv_Q_former3));
inv_Q4 = max(y_d - inv_threshold(4),min(y_d + inv_threshold(4),inv_Q_former4));
inv_Q5 = max(y_d - inv_threshold(5),min(y_d + inv_threshold(5),inv_Q_former5));
inv_Q6 = max(y_d - inv_threshold(6),min(y_d + inv_threshold(6),inv_Q_former6));
inv_Q7 = max(y_d - inv_threshold(7),min(y_d + inv_threshold(7),inv_Q_former7));
inv_Q8 = max(y_d - inv_threshold(8),min(y_d + inv_threshold(8),inv_Q_former8));
inv_Q9 = max(y_d - inv_threshold(9),min(y_d + inv_threshold(9),inv_Q_former9));
inv_Q10 = max(y_d - inv_threshold(10),min(y_d + inv_threshold(10),inv_Q_former10));
B = [inv_weigh(1).*inv_Q1,inv_weigh(2).*inv_Q2,inv_weigh(3).*inv_Q3,inv_weigh(4).*inv_Q4,inv_weigh(5).*inv_Q5,inv_weigh(6).*inv_Q6,inv_weigh(7).*inv_Q7,inv_weigh(8).*inv_Q8,inv_weigh(9).*inv_Q9,inv_weigh(10).*inv_Q10];
inv_PI = sum(B);
